simulink model "massspirngdamper"  (Simulink 8.4)
settings: Solver=ode45  StartTime=0.0  StopTime=10.0  RelTol=1e-3
settings Model: Creator=didichi  LastModifiedBy=didichi
settings DataIOCC: SignalLoggingSaveFormat=Dataset
settings OptimizationCC: ExpressionDepthLimit=128
settings DebuggingCC: UnderspecifiedInitializationDetection=Simplified  MergeDetectMultiDrivingBlocksExec=error  FcnCallInpInsideContextMsg=EnableAllAsError  StateNameClashWarn=none
settings GRTTargetCC: CombineOutputUpdateFcns=on  GRTInterface=off

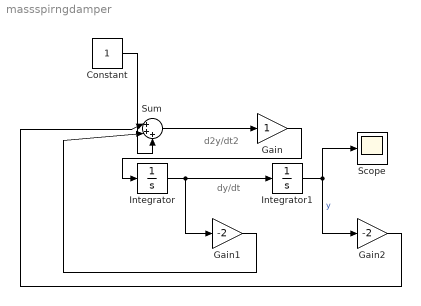
== system massspirngdamper ==
  note: dy/dt
  note: d2y/dt2
  Constant : Constant
  Gain : Gain
  Gain1 : Gain  Gain=-2
  Gain2 : Gain  Gain=-2
  Integrator : Integrator
  Integrator1 : Integrator
  Scope : Scope
  Sum : Sum  Inputs=|+++
  wires:
  Sum/1 -> Gain/1
  Integrator/1 -> Gain1/1, Integrator1/1
  Integrator1/1 -> Gain2/1, Scope/1  "y"
  Gain2/1 -> Sum/1
  Gain1/1 -> Sum/2
  Gain/1 -> Integrator/1
  Constant/1 -> Sum/3
